simulink model "distmodel_v6_LLSat"  (R2023b)
settings: Solver=FixedStepAuto  StartTime=0.0  StopTime=t_sim  FixedStep=TimeStep  RelTol=1e-3
values from neighbouring files (symbols this model uses):
  alt = 300    [main_disturbances.m]    (also in main_disturbances_LLSat.m = 275)
  angle_roll = pi/4    (= 0.785398163397)    [main_disturbances_LLSat.m]
  c = 299792458    [main_disturbances.m]    (also in main_disturbances_LLSat.m)
  Cd = 2.4    [SNAP_aero_CreateTorqueProfile.m]    (also in SNAP_aero_CreateTorqueProfile_LLSat.m = 2.5; SNAP_aero_CreateTorqueProfile_LLSat2.m = 2.5; main_disturbances.m; main_disturbances_LLSat.m = 2.5)
  D = [x_th-x_cog;y_th-y_cog;z_th-z_cog]/1e3    [momentumstorage.m]
  date_IGRF = [date.year,date.month,date.day]    [main_disturbances.m]    (also in main_disturbances_LLSat.m)
  F_s = 1367    [main_disturbances.m]    (also in main_disturbances_LLSat.m)
  inc = rad2deg(inc)    [main_disturbances.m]    (also in main_disturbances_LLSat.m)
  nmax = 2    [main_disturbances.m]    (also in main_disturbances_LLSat.m)
  nu = rad2deg(nu)    [main_disturbances.m]    (also in main_disturbances_LLSat.m)
  q = 0.6    [main_disturbances.m]    (also in main_disturbances_LLSat.m)
  RAAN = rad2deg(RAAN)    [main_disturbances.m]    (also in main_disturbances_LLSat.m)
  Use_IGRF = 0    [main_disturbances.m]    (also in main_disturbances_LLSat.m)
  w = find(volume(:,y,z) == 1)    [calc_torque_v1.m]    (also in calc_torque_v2.m; main_disturbances.m = rad2deg(w); main_disturbances_LLSat.m = rad2deg(w))
undefined symbols (not defined in the file or in its folder): date, DipoleMod, ecc, LLSataero, sat
libraries: vrlib x13, dspmathops x12, sharedtransform x10, aerolibutil x7, simulink_extras x4, matrix_library x2, aerolibconvert2 x1, aerolibatmos2 x1, aerolibobsolete x1
(part 2 of 2)

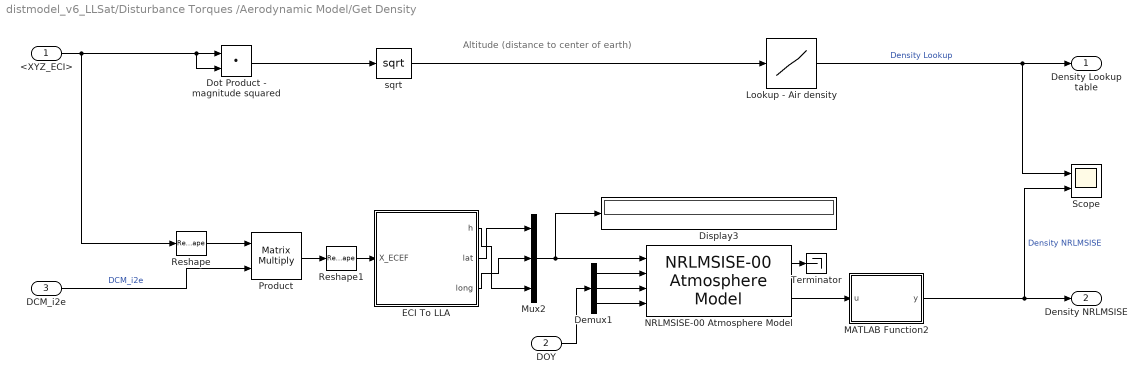
== system distmodel_v6_LLSat/Disturbance Torques /Aerodynamic Model/Get Density ==
  note: Altitude (distance to center of earth)
  <XYZ_ECI> : Inport
  DOY : Inport  Port=2
  "DCM_i2e " : Inport  Port=3
  Demux1 : Demux  Outputs=3
  Display3 : Display
  Dot Product - magnitude squared : DotProduct  OutDataTypeStr=Inherit: Inherit via internal rule
  ECI To LLA : MATLAB Function  TreatAsAtomicUnit=on
  Lookup - Air density : Lookup  InputValues=LLSataero.alt_range*1000 + 6378100  Table=LLSataero.av_density_vs_alt  SaturateOnIntegerOverflow=off
  MATLAB Function2 : MATLAB Function  TreatAsAtomicUnit=on
  Mux2 : Mux  Inputs=3
  NRLMSISE-00 Atmosphere Model : aerolibatmos2/NRLMSISE-00 Atmosphere Model  units=Metric (MKS)  lst_input=off  flux_ap_input=off  flags_input=Internal  flags=ones(1,23)  oxygen_in=on  action=Warning
  Product : Product  Multiplication=Matrix(*)
  Reshape : Reshape  OutputDimensionality=Row vector (2-D)
  Reshape1 : Reshape  OutputDimensionality=Row vector (2-D)
  Scope : Scope  NumInputPorts=2
  Terminator : Terminator
  sqrt : Math  Operator=sqrt  SignedPower=on
  Density Lookup table : Outport
  Density NRLMSISE : Outport  Port=2
  wires:
  Dot Product - magnitude squared/1 -> sqrt/1
  Lookup - Air density/1 -> Scope/1, Density Lookup table/1  "Density Lookup"
  sqrt/1 -> Lookup - Air density/1
  DOY/1 -> Demux1/1
  Demux1/1 -> NRLMSISE-00 Atmosphere Model/2
  Demux1/2 -> NRLMSISE-00 Atmosphere Model/3
  NRLMSISE-00 Atmosphere Model/2 -> MATLAB Function2/1(u)
  Demux1/3 -> NRLMSISE-00 Atmosphere Model/4
  Mux2/1 -> Display3/1, NRLMSISE-00 Atmosphere Model/1
  NRLMSISE-00 Atmosphere Model/1 -> Terminator/1
  MATLAB Function2/1(y) -> Scope/2, Density NRLMSISE/1  "Density NRLMSISE"
  Reshape/1 -> Product/1
  "DCM_i2e "/1 -> Product/2  "DCM_i2e"
  <XYZ_ECI>/1 -> Reshape/1, Dot Product - magnitude squared/1, Dot Product - magnitude squared/2
  Product/1 -> Reshape1/1
  ECI To LLA/2(lat) -> Mux2/1
  ECI To LLA/3(long) -> Mux2/2
  ECI To LLA/1(h) -> Mux2/3
  Reshape1/1 -> ECI To LLA/1(X_ECEF)

== system distmodel_v6_LLSat/Disturbance Torques /Solar Radiation Model/Calculate - Az & El Angle ==
  attitude : Inport
  sun unit ECI : Inport  Port=2
  Acos1 : Trigonometry  Operator=acos
  Atan1 : Trigonometry  Operator=atan
  Constant : Constant  Value=pi/2
  Demux : Demux  Outputs=3
  Divide : Product  Inputs=*/
  MATLAB Function : MATLAB Function  TreatAsAtomicUnit=on
  Rotation : Product  Multiplication=Matrix(*)  RndMeth=Zero
  Scope1 : Scope
  Scope2 : Scope
  Scope5 : Scope
  Scope6 : Scope  NumInputPorts=2
  Sum1 : Sum  Inputs=|+-
  El1 : Outport
  Az1 : Outport  Port=2
  wires:
  attitude/1 -> Rotation/1  "ECI to BRF"
  sun unit ECI/1 -> Rotation/2
  Rotation/1 -> Demux/1  "wind BRF"
  Demux/2 -> MATLAB Function/2(y), Scope5/1, Divide/1
  Atan1/1 -> Scope6/1, Az1/1
  Demux/1 -> Divide/2, MATLAB Function/1(x), Scope1/1
  Demux/3 -> MATLAB Function/3(z)
  Acos1/1 -> Scope2/1, Sum1/1  "Elevation"
  Sum1/1 -> Scope6/2, El1/1
  Constant/1 -> Sum1/2
  MATLAB Function/1(elevation) -> Acos1/1
  Divide/1 -> Atan1/1

== system distmodel_v6_LLSat/IGRF Computation block/Obtain B_ECI/Dipole Subsystem ==
  In1 : Inport
  Action Port : ActionPort  ActionPortLabel=else
  Bus Selector1 : BusSelector  OutputSignals=h,lat,long,DCM_i2e
  Dipole Model : Subsystem  AncestorBlock=DipoleModel/Dipole Model
  "B_ECI " : Outport  VectorParamsAs1DForOutWhenUnconnected=off
  wires:
  In1/1 -> Bus Selector1/1
  Bus Selector1/1 -> Dipole Model/1(h)  "<h>"
  Bus Selector1/2 -> Dipole Model/2("lat ")  "<lat>"
  Bus Selector1/3 -> Dipole Model/3(long)  "<long>"
  Bus Selector1/4 -> Dipole Model/4(ECI2ECEF_DCM)  "<DCM_i2e>"
  Dipole Model/1("B_ECI ") -> "B_ECI "/1

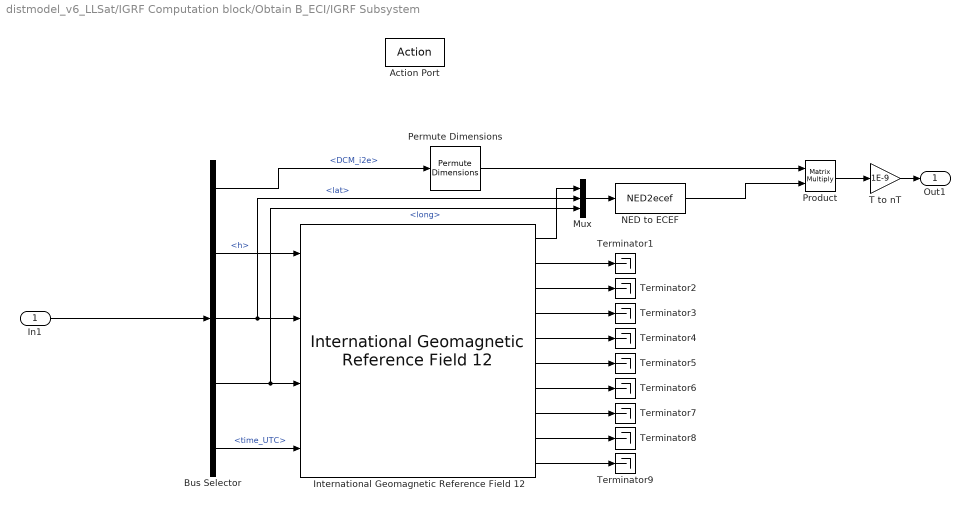
== system distmodel_v6_LLSat/IGRF Computation block/Obtain B_ECI/IGRF Subsystem ==
  In1 : Inport
  Action Port : ActionPort  ActionPortLabel=if(u1 > 0)
  Bus Selector : BusSelector  OutputSignals=DCM_i2e,h,lat,long,time_UTC
  International Geomagnetic Reference Field 12 : aerolibobsolete/International Geomagnetic Reference Field 12  units=Metric (MKS)  time_in=on  month=January  day=1  year=2020  action=None  sv_out=on
  Mux : Mux  Inputs=3
  NED to ECEF : MATLABFcn  MATLABFcn=NED2ecef  OutputDimensions=[3;1]  Output1D=off
  Permute Dimensions : PermuteDimensions
  Product : Product  Multiplication=Matrix(*)
  T to nT : Gain  Gain=1E-9
  Terminator{1..9} (9 alike) : Terminator
  Out1 : Outport  VectorParamsAs1DForOutWhenUnconnected=off
  wires:
  In1/1 -> Bus Selector/1
  Bus Selector/2 -> International Geomagnetic Reference Field 12/1  "<h>"
  T to nT/1 -> Out1/1
  Bus Selector/5 -> International Geomagnetic Reference Field 12/4  "<time_UTC>"
  Bus Selector/4 -> Mux/3, International Geomagnetic Reference Field 12/3  "<long>"
  Bus Selector/3 -> Mux/2, International Geomagnetic Reference Field 12/2  "<lat>"
  International Geomagnetic Reference Field 12/2 -> Terminator1/1
  International Geomagnetic Reference Field 12/10 -> Terminator9/1
  International Geomagnetic Reference Field 12/4 -> Terminator3/1
  International Geomagnetic Reference Field 12/5 -> Terminator4/1
  International Geomagnetic Reference Field 12/3 -> Terminator2/1
  International Geomagnetic Reference Field 12/1 -> Mux/1
  International Geomagnetic Reference Field 12/6 -> Terminator5/1
  International Geomagnetic Reference Field 12/8 -> Terminator7/1
  International Geomagnetic Reference Field 12/7 -> Terminator6/1
  International Geomagnetic Reference Field 12/9 -> Terminator8/1
  Bus Selector/1 -> Permute Dimensions/1  "<DCM_i2e>"
  Permute Dimensions/1 -> Product/1
  Product/1 -> T to nT/1
  Mux/1 -> NED to ECEF/1
  NED to ECEF/1 -> Product/2

== system distmodel_v6_LLSat/IGRF Computation block/Obtain B_ECI/Dipole Subsystem/Dipole Model ==
  h : Inport
  "lat " : Inport  Port=2
  long : Inport  Port=3
  ECI2ECEF_DCM : Inport  Port=4
  Bus Creator : BusCreator  Inputs=3
  Interpreted MATLAB Function : MATLABFcn  MATLABFcn=DipoleMod(u(1),u(2),u(3),date_IGRF,nmax)
  Permute Dimensions : PermuteDimensions
  Product : Product  Multiplication=Matrix(*)
  scaling from nT to T : Gain  Gain=1e-9
  "B_ECI " : Outport  VectorParamsAs1DForOutWhenUnconnected=off
  wires:
  Product/1 -> scaling from nT to T/1
  Permute Dimensions/1 -> Product/1
  ECI2ECEF_DCM/1 -> Permute Dimensions/1
  Bus Creator/1 -> Interpreted MATLAB Function/1
  "lat "/1 -> Bus Creator/2
  long/1 -> Bus Creator/3
  scaling from nT to T/1 -> "B_ECI "/1
  Interpreted MATLAB Function/1 -> Product/2
  h/1 -> Bus Creator/1

== matlab function distmodel_v6_LLSat/Disturbance Torques /Aerodynamic Model/Get Density/ECI To LLA ==
  data: X_ECEF input; h output; lat output; long output
function [h, lat, long] = fcn(X_ECEF)
    % h = 0;
    % lat = 0;
    % long = 0;
%[lat, long, h] = ecef2geod(X_ECEF(1),X_ECEF(2),X_ECEF(3));
[ans] = ecef2geod([X_ECEF(1),X_ECEF(2),X_ECEF(3)]);
lat=ans(1);
long=ans(2);
h=ans(3);

== matlab function distmodel_v6_LLSat/IGRF Computation block/ECI To LLA ==
  data: X_ECEF input; h output; lat output; long output
function [h, lat, long] = fcn(X_ECEF)
[ans] = ecef2geod([X_ECEF(1),X_ECEF(2),X_ECEF(3)]);
lat=ans(1);
long=ans(2);
h=ans(3);

== matlab function distmodel_v6_LLSat/Disturbance Torques /Solar Radiation Model/Calculate - Az & El Angle/MATLAB Function ==
  data: x input; elevation output; y input; z input
function elevation = fcn(x,y,z)

elevation = z/sqrt(x^2 + y^2 + z^2);

== matlab function distmodel_v6_LLSat/Disturbance Torques /Aerodynamic Model/Get Density/MATLAB Function2 ==
  data: u input; y output
function y = fcn(u)
y = u(6);

== matlab function distmodel_v6_LLSat/Time propagator/UTC to JD ==
  data: Time_UTC input; JD output
function JD = fcn(Time_UTC)

% JD = juliandate(Time_UTC);
JD = Dt2jD(Time_UTC);

== matlab function distmodel_v6_LLSat/Time propagator/JD to UTC ==
  data: JD input; Time_UTC output
function Time_UTC = fcn(JD)
    coder.extrinsic('datetime','datevec');
    Time_UTC = [0,0,0,0,0,0];
Time_UTC =  datevec(datetime(JD,'convertfrom','juliandate'));

== matlab function distmodel_v6_LLSat/Disturbance Torques /Aerodynamic Model/Calculate - Az & El Angle/MATLAB Function ==
  data: x input; elevation output; y input; z input
function elevation = fcn(x,y,z)

elevation = z/sqrt(x^2 + y^2 + z^2);

== matlab function distmodel_v6_LLSat/Time propagator/MATLAB Function ==
  data: t input; Y output; DOY output; S output
function [Y, DOY, S] = DOY(t)
Y = 2022 + fix(t/31557600);
DOY = 1+fix((t-floor(t/31557600)*31557600)/86400);
S = t - fix(t/31557600)*31557600 - (DOY-1)*86400;
